simulink model "TPPFC_fast_PI"  (R2024a)
settings: Solver=FixedStepDiscrete  StartTime=0.0  StopTime=0.6  FixedStep=Ts_Power  RelTol=1e-3  AbsTol=1e-3  EnableMultiTasking=on
values from neighbouring files (symbols this model uses):
  C_PFC = 2240e-6    (= 0.00224)    [TPPFC_fast_PI_data.m]    (also in TPPFC_me_fast_PI_data.m)
  Fnom = 50    [TPPFC_fast_PI_data.m]    (also in TPPFC_me_fast_PI_data.m)
  K_ii = K_ip/T_ii    [TPPFC_fast_PI_data.m]    (also in TPPFC_me_fast_PI_data.m)
  K_ip = 2*pi*f_ci*L_PFC/sqrt(2)/Vnom_dc    [TPPFC_fast_PI_data.m]    (also in TPPFC_me_fast_PI_data.m)
  K_vi = K_vp/T_vi    (= 14.738609239)    [TPPFC_fast_PI_data.m]    (also in TPPFC_me_fast_PI_data.m)
  K_vp = 2*pi*f_cv*C_PFC*Vnom_dc/Vnom_ac    (= 0.234572251468)    [TPPFC_fast_PI_data.m]    (also in TPPFC_me_fast_PI_data.m)
  L_PFC = 400e-6    (= 0.0004)    [TPPFC_fast_PI_data.m]    (also in TPPFC_me_fast_PI_data.m)
  RL_PFC = 40e-3    (= 0.04)    [TPPFC_fast_PI_data.m]    (also in TPPFC_me_fast_PI_data.m)
  Ro = 24.24    [TPPFC_fast_PI_data.m]    (also in TPPFC_me_fast_PI_data.m)
  Ts_Control = 10e-6    (= 1e-05)    [TPPFC_fast_PI_data.m]    (also in TPPFC_me_fast_PI_data.m)
  Ts_Power = 50e-9    (= 5e-08)    [TPPFC_fast_PI_data.m]    (also in TPPFC_me_fast_PI_data.m)
  Vnom_ac = 240    [TPPFC_fast_PI_data.m]    (also in TPPFC_me_fast_PI_data.m)
  Vnom_dc = 400    [TPPFC_fast_PI_data.m]    (also in TPPFC_me_fast_PI_data.m)
libraries: spsMosfetLib x4, spsSeriesRLCBranchLib x4, spsMeanLib x3, slpidlib x2, spsCurrentMeasurementLib x2, spsVoltageMeasurementLib x2, spsACVoltageSourceLib x1, spsPLLLib x1, spsPWMGeneratorDCDCLib x1, spsIdealSwitchLib x1, spsFourierLib x1, spsPowerLib x1
settings Model: SimulationMode=accelerator  Creator=LWYohann  LastModifiedBy=LWYohann
settings SolverCC: AutoScaleAbsTol=off  AlgebraicLoopSolver=TrustRegion  MaxZcPerStep=1
settings DebuggingCC: UnconnectedInputMsg=warning  UnconnectedOutputMsg=warning  UnconnectedLineMsg=warning  SymbolicDimsDataTypeCodeGenerationDiagnostic=none
settings ModelReferenceCC: EnableRefExpFcnMdlSchedulingChecks=on
settings SFSimCC: CustomCodeUndefinedFunction=UseInterfaceOnly
settings RTWCC: GPUComputeCapability=3.5  DLArmComputeVersion=19.05
settings SimscapeCC: ExplicitSolverDiagnosticOptions=none  SimscapeLogType=all  SimscapeLogSimulationStatistics=on  SimscapeLogDataHistory=10000

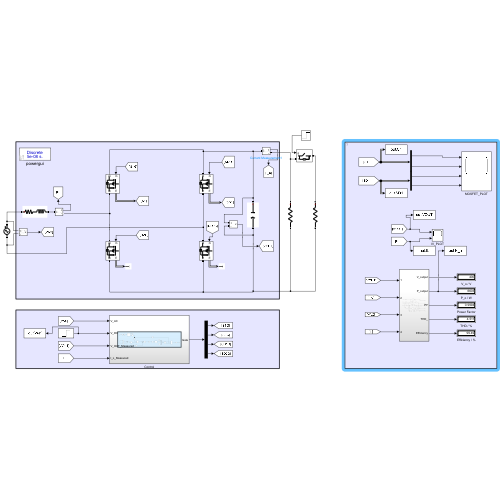
[thumbnail: Simulink's stored preview of the top-level diagram]
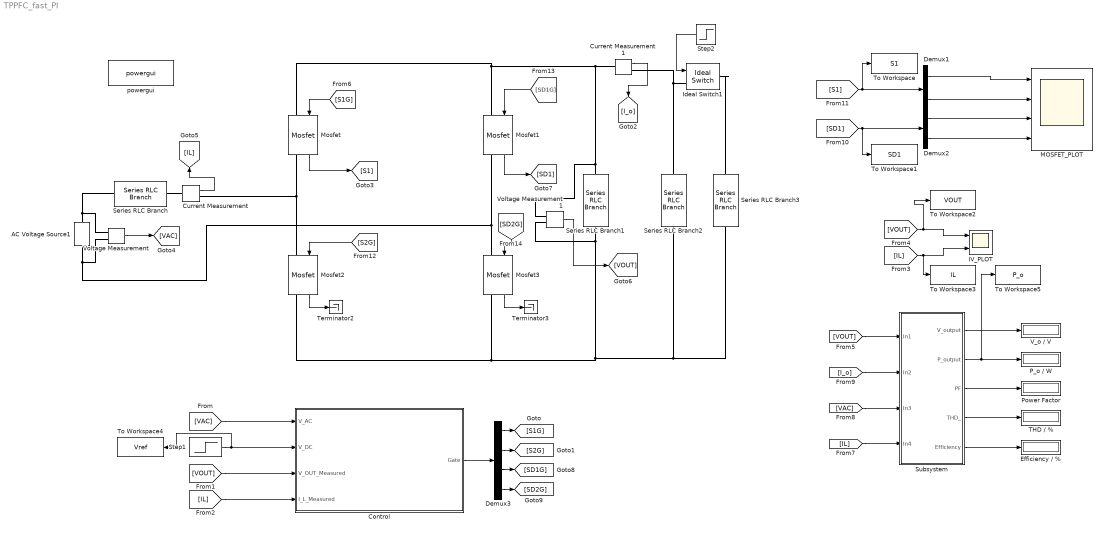
== system TPPFC_fast_PI ==
  AC Voltage Source1 : spsACVoltageSourceLib/AC Voltage Source  Amplitude=Vnom_ac*sqrt(2)  Phase=0  Frequency=Fnom  SampleTime=Ts_Power  Measurements=None  BusType=swing  Pref=10e3  Qref=0  Qmin=-inf  Qmax=+inf
  Control : Subsystem
  Current Measurement : spsCurrentMeasurementLib/Current Measurement  PhasorSimulation=off  OutputType=Complex  PSBequivalent=0
  Current Measurement1 : spsCurrentMeasurementLib/Current Measurement  PhasorSimulation=off  OutputType=Complex  PSBequivalent=0
  Demux1 : Demux  Outputs=2
  Demux2 : Demux  Outputs=2
  Demux3 : Demux
  Efficiency / % : Display
      settings: Decimation=100
  IV_PLOT : Scope  NumInputPorts=2
  Ideal Switch1 : spsIdealSwitchLib/Ideal Switch  Ron=0.001  Lon=0  IC=0  Rs=1e5  Cs=inf  Measurements=off
  MOSFET_PLOT : Scope  NumInputPorts=4
  Mosfet{,1..3} (4 alike) : spsMosfetLib/Mosfet  Ron=Ron_FET  Lon=0  Rd=Ron_Diode  Vfd=Vf  IC=0  Rs=1e6  Cs=inf  Measurements=on
  P_o / W : Display
  Power Factor : Display
  Series RLC Branch : spsSeriesRLCBranchLib/Series RLC Branch  LConnTagsString=__new0  RConnTagsString=__new0  BranchType=RL  Resistance=RL_PFC  Inductance=L_PFC  SetiL0=off  InitialCurrent=0  Capacitance=1e-6  Setx0=off  InitialVoltage=0  Measurements=None
  Series RLC Branch1 : spsSeriesRLCBranchLib/Series RLC Branch  LConnTagsString=__new0  RConnTagsString=__new0  BranchType=C  Resistance=RL_PFC  Inductance=L_PFC  SetiL0=off  InitialCurrent=0  Capacitance=C_PFC  Setx0=on  InitialVoltage=375  Measurements=None
  Series RLC Branch2 : spsSeriesRLCBranchLib/Series RLC Branch  LConnTagsString=__new0  RConnTagsString=__new0  BranchType=R  Resistance=2*Ro  Inductance=L_PFC  SetiL0=off  InitialCurrent=0  Capacitance=C_PFC  Setx0=off  InitialVoltage=0  Measurements=None
  Series RLC Branch3 : spsSeriesRLCBranchLib/Series RLC Branch  LConnTagsString=__new0  RConnTagsString=__new0  BranchType=R  Resistance=2*Ro  Inductance=L_PFC  SetiL0=off  InitialCurrent=0  Capacitance=C_PFC  Setx0=off  InitialVoltage=0  Measurements=None
  Step1 : Step  Time=0.2  Before=350  After=Vnom_dc  SampleTime=Ts_Power
  Step2 : Step  Time=0.4  SampleTime=Ts_Power
  Subsystem : Subsystem
  THD / % : Display
  Terminator2 : Terminator
  Terminator3 : Terminator
  To Workspace : ToWorkspace  VariableName=S1  SaveFormat=Structure With Time  SampleTime=Ts_Control
  To Workspace1 : ToWorkspace  VariableName=SD1  SaveFormat=Structure With Time  SampleTime=Ts_Control
  To Workspace2 : ToWorkspace  VariableName=VOUT  SaveFormat=Structure With Time  SampleTime=Ts_Control
  To Workspace3 : ToWorkspace  VariableName=IL  SaveFormat=Structure With Time  SampleTime=Ts_Control
  To Workspace4 : ToWorkspace  VariableName=Vref  SaveFormat=Structure With Time  SampleTime=Ts_Control
  To Workspace5 : ToWorkspace  VariableName=P_o  SaveFormat=Structure With Time  SampleTime=Ts_Control
  V_o / V : Display
  Voltage Measurement : spsVoltageMeasurementLib/Voltage Measurement  PhasorSimulation=off  OutputType=Complex  PSBequivalent=0
  Voltage Measurement1 : spsVoltageMeasurementLib/Voltage Measurement  PhasorSimulation=off  OutputType=Complex  PSBequivalent=0
  powergui : spspowerguiLib/powergui  Priority=1  SimulationMode=Discrete  SampleTime=Ts_Power  frequency=60  Iterations=50  frequencyindice=0  Pbase=100e6  ErrMax=1e-4  UnitsV=kV  UnitsW=MW  buscounter=0  FunctionMessages=off  echomessages=off  EnableUseOfTLC=off  CurrentSourceSwitches=off  DisableSnubberDevices=off  DisableRonSwitches=off  DisableVfSwitches=off  DisplayEquations=off  AutomaticDiscreteSolvers=off  SolverType=Tustin/Backward Euler (TBE)  Interpol=off  ExternalGateDelay=off  methode=off  Ts=100  x0status=blocks  SPID=on  SwTol=0  HookPort=off  NonlinearTolerance=1e-4  nMaxIteration=100  ContinueOnMaxIteration=off  RestoreLinks=warning  ResistiveCurrentMeasurement=off  Frange=[0:2:500]  Ylog=off  Xlog=on  ShowGrid=off  save=off  variable=ZData  structure=0  ZoomFFT=off  StartTime=0.0  cycles=1  DisplayStyle=1  fundamental=60  FreqAxis=off  MaxFrequency=1000  frequencyindicesteady=1  RmsSteady=1  display=off
  wires:
  Voltage Measurement/1 -> [VAC]
  Current Measurement/1 -> [IL]
  Voltage Measurement1/1 -> [VOUT]
  [IL] -> To Workspace3/1, IV_PLOT/2
  [VOUT] -> To Workspace2/1, IV_PLOT/1
  Current Measurement1/1 -> [I_o]
  Mosfet1/1 -> [SD1]
  Mosfet3/1 -> Terminator3/1
  Mosfet/1 -> [S1]
  Mosfet2/1 -> Terminator2/1
  [S1] -> To Workspace/1, Demux1/1
  Demux1/1 -> MOSFET_PLOT/1
  Demux1/2 -> MOSFET_PLOT/2
  Demux2/1 -> MOSFET_PLOT/3
  [SD1] -> To Workspace1/1, Demux2/1
  Demux2/2 -> MOSFET_PLOT/4
  Demux3/1 -> [S1G]
  Demux3/2 -> [S2G]
  Demux3/3 -> [SD1G]
  Demux3/4 -> [SD2G]
  [S1G] -> Mosfet/1
  [S2G] -> Mosfet2/1
  [SD1G] -> Mosfet1/1
  [SD2G] -> Mosfet3/1
  [VAC] -> Control/1(V_AC)
  Step1/1 -> To Workspace4/1, Control/2(V_DC)
  [VOUT] -> Control/3(V_OUT_Measured)
  [IL] -> Control/4(I_L_Measured)
  Control/1(Gate) -> Demux3/1
  [VOUT] -> Subsystem/1(In1)
  [I_o] -> Subsystem/2(In2)
  [VAC] -> Subsystem/3(In3)
  [IL] -> Subsystem/4(In4)
  Subsystem/1(V_output) -> V_o / V/1
  Subsystem/2(P_output) -> P_o / W/1, To Workspace5/1
  Subsystem/3(PF) -> Power Factor/1
  Subsystem/4(THD_) -> THD / %/1
  Subsystem/5(Efficiency) -> Efficiency / %/1
  Step2/1 -> Ideal Switch1/1
  connections:
  Series RLC Branch/LConn1 -- Voltage Measurement/LConn1 -- AC Voltage Source1/RConn1
  Mosfet2/RConn1 -- Mosfet3/RConn1 -- Series RLC Branch3/RConn1 -- Series RLC Branch2/RConn1 -- Series RLC Branch1/RConn1 -- Voltage Measurement1/LConn2
  Current Measurement/LConn1 -- Series RLC Branch/RConn1
  Mosfet/RConn1 -- Current Measurement/RConn1 -- Mosfet2/LConn1
  Mosfet/LConn1 -- Voltage Measurement1/LConn1 -- Series RLC Branch1/LConn1 -- Current Measurement1/LConn1 -- Mosfet1/LConn1
  Mosfet3/LConn1 -- Mosfet1/RConn1 -- Voltage Measurement/LConn2 -- AC Voltage Source1/LConn1
  Current Measurement1/RConn1 -- Ideal Switch1/LConn1 -- Series RLC Branch2/LConn1
  Ideal Switch1/RConn1 -- Series RLC Branch3/LConn1

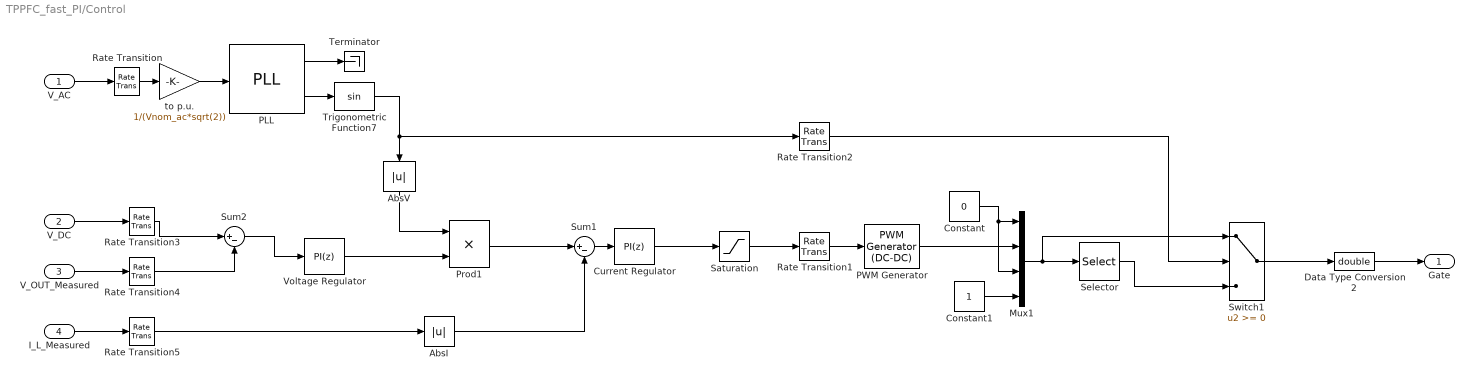
== system TPPFC_fast_PI/Control ==
  V_AC : Inport
  V_DC : Inport  Port=2
  V_OUT_Measured : Inport  Port=3
  I_L_Measured : Inport  Port=4
  AbsI : Abs  SaturateOnIntegerOverflow=off
  AbsV : Abs  SaturateOnIntegerOverflow=off
  Constant : Constant  Value=0
  Constant1 : Constant
  Current Regulator : slpidlib/PID Controller  Controller=PI  Form=Parallel  TimeDomain=Discrete-time  UseExternalTs=off  SampleTime=Ts_Control  IntegratorMethod=Forward Euler  FilterMethod=Forward Euler  ControllerParametersSource=internal  P=K_ip  I=K_ii  UseKiTs=off  D=0  UseExternalDerivativeSource=off  N=100  UseFilter=on  TunerSelectOption=Transfer Function Based (PID Tuner App)  InitialConditionSource=internal  InitialConditionForIntegrator=0  InitialConditionForFilter=0  DifferentiatorICPrevScaledInput=0  ExternalReset=none  TrackingMode=off  Kt=1  LimitOutput=off  SatLimitsSource=internal  UpperSaturationLimit=inf  LowerSaturationLimit=-inf  LinearizeAsGain=on  AntiWindupMode=none  Kb=1  LimitIntegrator=off  UpperIntegratorSaturationLimit=inf  LowerIntegratorSaturationLimit=-inf  POutMin=[]  POutMax=[]  IOutMin=[]  IOutMax=[]  DOutMin=[]  DOutMax=[]  NOutMin=[]  NOutMax=[]  SumOutMin=[]  SumOutMax=[]  SaturationOutMin=[]  SaturationOutMax=[]  PParamMin=[]  PParamMax=[]  IParamMin=[]  IParamMax=[]  DParamMin=[]  DParamMax=[]  NParamMin=[]  NParamMax=[]  KbParamMin=[]  KbParamMax=[]  KtParamMin=[]  KtParamMax=[]  KbOutMin=[]  KbOutMax=[]  KtOutMin=[]  KtOutMax=[]  IntegratorOutMin=[]  IntegratorOutMax=[]  FilterOutMin=[]  FilterOutMax=[]  SumI1OutMin=[]  SumI1OutMax=[]  SumI2OutMin=[]  SumI2OutMax=[]  SumI3OutMin=[]  SumI3OutMax=[]  SumI4OutMin=[]  SumI4OutMax=[]  SumDOutMin=[]  SumDOutMax=[]  DifferentiatorOutMin=[]  DifferentiatorOutMax=[]  FilterDiffOutCoefMin=[]  FilterDiffOutCoefMax=[]  ReciprocalOutMin=[]  ReciprocalOutMax=[]  SumDenOutMin=[]  SumDenOutMax=[]  SumNumOutMin=[]  SumNumOutMax=[]  DivideOutMin=[]  DivideOutMax=[]  UdiffTsProdOutMin=[]  UdiffTsProdOutMax=[]  NTsProdOutMin=[]  NTsProdOutMax=[]  UintegralTsProdOutMin=[]  UintegralTsProdOutMax=[]  UngainTsProdOutMin=[]  UngainTsProdOutMax=[]  ClampingZeroOutDataTypeStr=Inherit: Inherit via back propagation  ClampingZeroOutMin=[]  ClampingZeroOutMax=[]  FilterDenConstantOutDataTypeStr=Inherit: Inherit via back propagation  FilterDenConstantOutMin=[]  FilterDenConstantOutMax=[]  PCopyOutDataTypeStr=Inherit: Inherit via back propagation  PCopyOutMin=[]  PCopyOutMax=[]  NCopyOutDataTypeStr=Inherit: Inherit via back propagation  NCopyOutMin=[]  NCopyOutMax=[]  IntegratorContinuousStateAttributes=''  IntegratorStateMustResolveToSignalObject=off  IntegratorRTWStateStorageClass=Auto  FilterContinuousStateAttributes=''  FilterStateMustResolveToSignalObject=off  FilterRTWStateStorageClass=Auto  ParallelPVariant=InternalParameters  IdealPVariant=Disabled  IVariant=InternalParameters  DVariant=Disabled  IntegratorVariant=Discrete  SatVariant=Disabled  AWVariant=Passthrough  PCopyVariant=Disabled  TRVariant=Disabled  FdbkBlocksVariant=Forward  IdealPFdbkVariant=Disabled  SatFdbkVariant=Disabled  DerivativeFilterVariant=Disabled  NVariant=Disabled  NCopyVariant=Disabled_SignalSpec  FilterICVariant=Disabled  IntegratorICVariant=InternalICs  ExternalResetVariant=Disabled  TRSumVariant=Passthrough  SumFdbkVariant=Disabled  SumVariant=Sum_PI  TsampFilterVariant=InternalTs  TsampNgainVariant=Passthrough  TsampIntegralVariant=Disabled_SignalSpec  ExternalSaturationOutDataTypeStr=Inherit: Same as second input  DerivativeSourceVariant=Disabled
  Data Type Conversion2 : DataTypeConversion  OutDataTypeStr=double  SaturateOnIntegerOverflow=off  RndMeth=Floor
  Mux1 : Mux
  PLL : spsPLLLib/PLL  Fmin=0.9*Fnom  Par_Init=[0, Fnom]  ParK=[180, 3200, 1]  TcD=1e-4  MaxRateChangeFreq=12  FilterCutOffFreq=25  Ts=Ts_Control  AGC=on
  PWM Generator : spsPWMGeneratorDCDCLib/PWM Generator (DC-DC)  Fsw=Fsw  Ts=Ts_Power
  Prod1 : Product
  Rate Transition{,3..5} (4 alike) : RateTransition  OutPortSampleTime=Ts_Control
  Rate Transition1 : RateTransition  OutPortSampleTime=Ts_Power
  Rate Transition2 : RateTransition  OutPortSampleTime=Ts_Power
  Saturation : Saturate  UpperLimit=1  LowerLimit=0
  Selector : Selector  InputPortWidth=4  IndexOptions=Index vector (dialog)  Indices=[2 1 4 3]  OutputSizes=1
  Sum1 : Sum  Inputs=|+-
  Sum2 : Sum  Inputs=|+-
  Switch1 : Switch  SaturateOnIntegerOverflow=off  InputSameDT=off
  Terminator : Terminator
  Trigonometric Function7 : Trigonometry
  Voltage Regulator : slpidlib/PID Controller  Controller=PI  Form=Parallel  TimeDomain=Discrete-time  UseExternalTs=off  SampleTime=Ts_Control  IntegratorMethod=Forward Euler  FilterMethod=Forward Euler  ControllerParametersSource=internal  P=K_vp  I=K_vi  UseKiTs=off  D=0  UseExternalDerivativeSource=off  N=100  UseFilter=on  TunerSelectOption=Transfer Function Based (PID Tuner App)  InitialConditionSource=internal  InitialConditionForIntegrator=0  InitialConditionForFilter=0  DifferentiatorICPrevScaledInput=0  ExternalReset=none  TrackingMode=off  Kt=1  LimitOutput=off  SatLimitsSource=internal  UpperSaturationLimit=inf  LowerSaturationLimit=-inf  LinearizeAsGain=on  AntiWindupMode=none  Kb=1  LimitIntegrator=off  UpperIntegratorSaturationLimit=inf  LowerIntegratorSaturationLimit=-inf  POutMin=[]  POutMax=[]  IOutMin=[]  IOutMax=[]  DOutMin=[]  DOutMax=[]  NOutMin=[]  NOutMax=[]  SumOutMin=[]  SumOutMax=[]  SaturationOutMin=[]  SaturationOutMax=[]  PParamMin=[]  PParamMax=[]  IParamMin=[]  IParamMax=[]  DParamMin=[]  DParamMax=[]  NParamMin=[]  NParamMax=[]  KbParamMin=[]  KbParamMax=[]  KtParamMin=[]  KtParamMax=[]  KbOutMin=[]  KbOutMax=[]  KtOutMin=[]  KtOutMax=[]  IntegratorOutMin=[]  IntegratorOutMax=[]  FilterOutMin=[]  FilterOutMax=[]  SumI1OutMin=[]  SumI1OutMax=[]  SumI2OutMin=[]  SumI2OutMax=[]  SumI3OutMin=[]  SumI3OutMax=[]  SumI4OutMin=[]  SumI4OutMax=[]  SumDOutMin=[]  SumDOutMax=[]  DifferentiatorOutMin=[]  DifferentiatorOutMax=[]  FilterDiffOutCoefMin=[]  FilterDiffOutCoefMax=[]  ReciprocalOutMin=[]  ReciprocalOutMax=[]  SumDenOutMin=[]  SumDenOutMax=[]  SumNumOutMin=[]  SumNumOutMax=[]  DivideOutMin=[]  DivideOutMax=[]  UdiffTsProdOutMin=[]  UdiffTsProdOutMax=[]  NTsProdOutMin=[]  NTsProdOutMax=[]  UintegralTsProdOutMin=[]  UintegralTsProdOutMax=[]  UngainTsProdOutMin=[]  UngainTsProdOutMax=[]  ClampingZeroOutDataTypeStr=Inherit: Inherit via back propagation  ClampingZeroOutMin=[]  ClampingZeroOutMax=[]  FilterDenConstantOutDataTypeStr=Inherit: Inherit via back propagation  FilterDenConstantOutMin=[]  FilterDenConstantOutMax=[]  PCopyOutDataTypeStr=Inherit: Inherit via back propagation  PCopyOutMin=[]  PCopyOutMax=[]  NCopyOutDataTypeStr=Inherit: Inherit via back propagation  NCopyOutMin=[]  NCopyOutMax=[]  IntegratorContinuousStateAttributes=''  IntegratorStateMustResolveToSignalObject=off  IntegratorRTWStateStorageClass=Auto  FilterContinuousStateAttributes=''  FilterStateMustResolveToSignalObject=off  FilterRTWStateStorageClass=Auto  ParallelPVariant=InternalParameters  IdealPVariant=Disabled  IVariant=InternalParameters  DVariant=Disabled  IntegratorVariant=Discrete  SatVariant=Disabled  AWVariant=Passthrough  PCopyVariant=Disabled  TRVariant=Disabled  FdbkBlocksVariant=Forward  IdealPFdbkVariant=Disabled  SatFdbkVariant=Disabled  DerivativeFilterVariant=Disabled  NVariant=Disabled  NCopyVariant=Disabled_SignalSpec  FilterICVariant=Disabled  IntegratorICVariant=InternalICs  ExternalResetVariant=Disabled  TRSumVariant=Passthrough  SumFdbkVariant=Disabled  SumVariant=Sum_PI  TsampFilterVariant=InternalTs  TsampNgainVariant=Passthrough  TsampIntegralVariant=Disabled_SignalSpec  ExternalSaturationOutDataTypeStr=Inherit: Same as second input  DerivativeSourceVariant=Disabled
  to p.u. : Gain  Gain=1/(Vnom_ac*sqrt(2))
  Gate : Outport
  wires:
  Rate Transition4/1 -> Sum2/2
  Constant/1 -> Mux1/3, Mux1/1
  Sum2/1 -> Voltage Regulator/1
  Sum1/1 -> Current Regulator/1
  V_DC/1 -> Rate Transition3/1
  V_AC/1 -> Rate Transition/1
  Rate Transition3/1 -> Sum2/1
  AbsI/1 -> Sum1/2
  Prod1/1 -> Sum1/1
  Rate Transition/1 -> to p.u./1
  Rate Transition2/1 -> Switch1/2
  PLL/2 -> Trigonometric Function7/1
  Trigonometric Function7/1 -> AbsV/1, Rate Transition2/1
  Switch1/1 -> Data Type Conversion2/1
  Mux1/1 -> Switch1/1, Selector/1
  Current Regulator/1 -> Saturation/1
  Voltage Regulator/1 -> Prod1/2
  V_OUT_Measured/1 -> Rate Transition4/1
  Rate Transition5/1 -> AbsI/1
  I_L_Measured/1 -> Rate Transition5/1
  Saturation/1 -> Rate Transition1/1
  Rate Transition1/1 -> PWM Generator/1
  Data Type Conversion2/1 -> Gate/1
  PWM Generator/1 -> Mux1/2
  Constant1/1 -> Mux1/4
  to p.u./1 -> PLL/1
  PLL/1 -> Terminator/1
  AbsV/1 -> Prod1/1
  Selector/1 -> Switch1/3

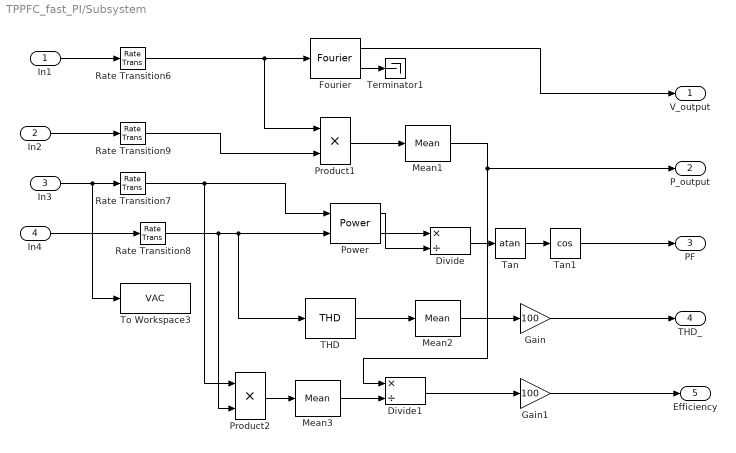
== system TPPFC_fast_PI/Subsystem ==
  In1 : Inport
  In2 : Inport  Port=2
  In3 : Inport  Port=3
  In4 : Inport  Port=4
  Divide : Product  Inputs=*/
  Divide1 : Product  Inputs=*/
  Fourier : spsFourierLib/Fourier  Freq=Fnom  n=0  InInit=[0, 0]  Ts=Ts_Control
  Gain : Gain  Gain=100
  Gain1 : Gain  Gain=100
  Mean1 : spsMeanLib/Mean  Freq=Fnom  Vinit=0  Ts=Ts_Control
  Mean2 : spsMeanLib/Mean  Freq=Fnom  Vinit=0  Ts=Ts_Control
  Mean3 : spsMeanLib/Mean  Freq=Fnom  Vinit=0  Ts=Ts_Control
  Power : spsPowerLib/Power  Freq=Fnom  Vinit=[1, 0]  Iinit=[1, 0]  Ts=Ts_Control
  Product1 : Product
  Product2 : Product
  Rate Transition{6..9} (4 alike) : RateTransition  OutPortSampleTime=Ts_Control
  THD : spsTHDLib/THD  Freq=Fnom  Ts=Ts_Control
  Tan : Trigonometry  Operator=atan
  Tan1 : Trigonometry  Operator=cos
  Terminator1 : Terminator
  To Workspace3 : ToWorkspace  VariableName=VAC  SaveFormat=Structure With Time  SampleTime=Ts_Control
  V_output : Outport
  P_output : Outport  Port=2
  PF : Outport  Port=3
  THD_ : Outport  Port=4
  Efficiency : Outport  Port=5
  wires:
  Fourier/2 -> Terminator1/1
  Product1/1 -> Mean1/1
  Rate Transition8/1 -> Product2/2, THD/1, Power/2
  Power/2 -> Divide/1
  Product2/1 -> Mean3/1
  Tan/1 -> Tan1/1
  THD/1 -> Mean2/1
  Mean3/1 -> Divide1/2
  Rate Transition6/1 -> Product1/1, Fourier/1
  Power/1 -> Divide/2
  Rate Transition9/1 -> Product1/2
  Divide/1 -> Tan/1
  Rate Transition7/1 -> Product2/1, Power/1
  Mean1/1 -> P_output/1, Divide1/1
  In3/1 -> To Workspace3/1, Rate Transition7/1
  Mean2/1 -> Gain/1
  Divide1/1 -> Gain1/1
  In2/1 -> Rate Transition9/1
  In1/1 -> Rate Transition6/1
  Fourier/1 -> V_output/1
  Tan1/1 -> PF/1
  In4/1 -> Rate Transition8/1
  Gain/1 -> THD_/1
  Gain1/1 -> Efficiency/1
